simulink model "Automated_IrrigationControlSystem"  (R2023a)
settings: Solver=VariableStepAuto  StartTime=0.0  StopTime=10  MaxStep=1e-3  RelTol=1e-3
libraries: simulink x2
settings Model: Creator=eslam  LastModifiedBy=eslam

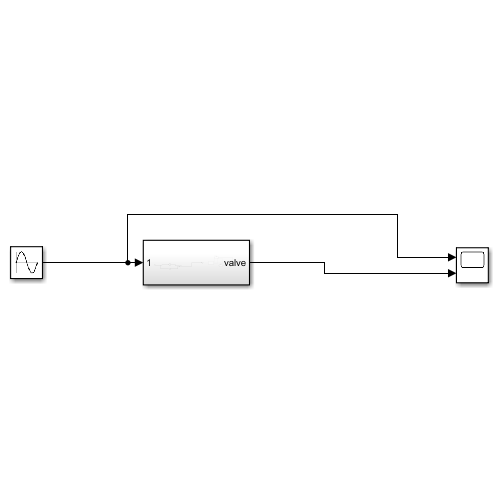
[thumbnail: Simulink's stored preview of the top-level diagram]
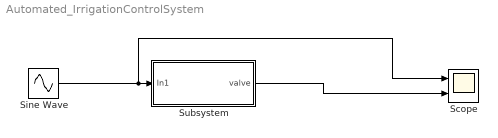
== system Automated_IrrigationControlSystem ==
  Scope : Scope  NumInputPorts=2
  Sine Wave : Sin  Amplitude=88  SampleTime=0
  Subsystem : Subsystem
  wires:
  Sine Wave/1 -> Scope/1, Subsystem/1(In1)
  Subsystem/1(" valve") -> Scope/2

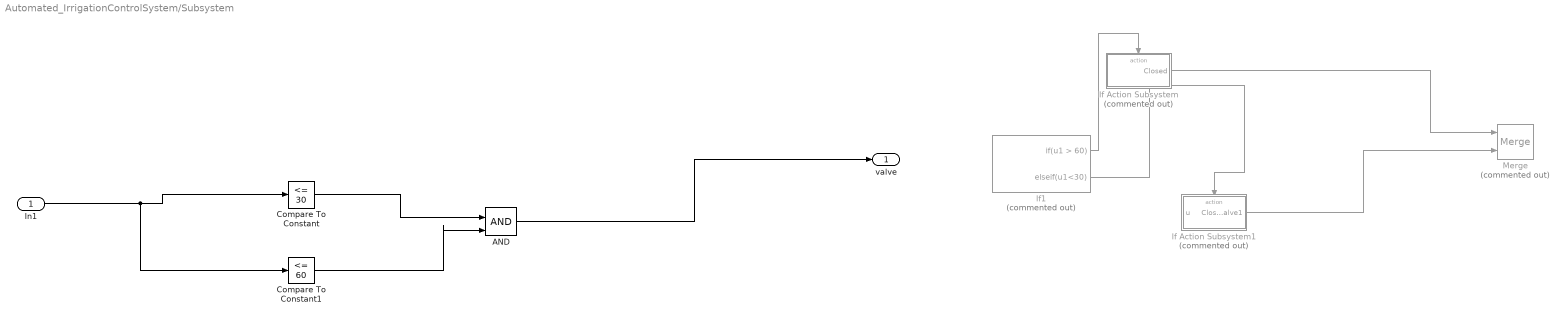
== system Automated_IrrigationControlSystem/Subsystem ==
  In1 : Inport
  AND : Logic  IconShape=distinctive  AllPortsSameDT=off  OutDataTypeStr=boolean
  Compare To Constant : simulink/Logic and Bit Operations/Compare To Constant  relop=<=  const=30  OutDataTypeStr=boolean
  Compare To Constant1 : simulink/Logic and Bit Operations/Compare To Constant  relop=<=  const=60  OutDataTypeStr=boolean
  If Action Subsystem : Subsystem  Commented=on  TreatAsAtomicUnit=on
  If Action Subsystem1 : Subsystem  Commented=on  TreatAsAtomicUnit=on
  If1 : If  Commented=on  IfExpression=u1 > 60  ElseIfExpressions=u1<30  ShowElse=off
  Merge : Merge  Commented=on
  " valve" : Outport
  wires:
  If1/1 -> If Action Subsystem/Action
  If1/2 -> If Action Subsystem1/Action
  If Action Subsystem1/1(Closed valve1) -> Merge/2
  If Action Subsystem/1(Closed) -> Merge/1
  Compare To Constant/1 -> AND/1
  Compare To Constant1/1 -> AND/2
  AND/1 -> " valve"/1
  In1/1 -> Compare To Constant1/1, Compare To Constant/1

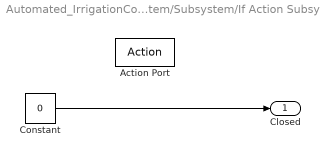
== system Automated_IrrigationControlSystem/Subsystem/If Action Subsystem ==
  Action Port : ActionPort  ActionPortLabel=if(u1 > 60)
  Constant : Constant  Value=0
  Closed : Outport
  wires:
  Constant/1 -> Closed/1

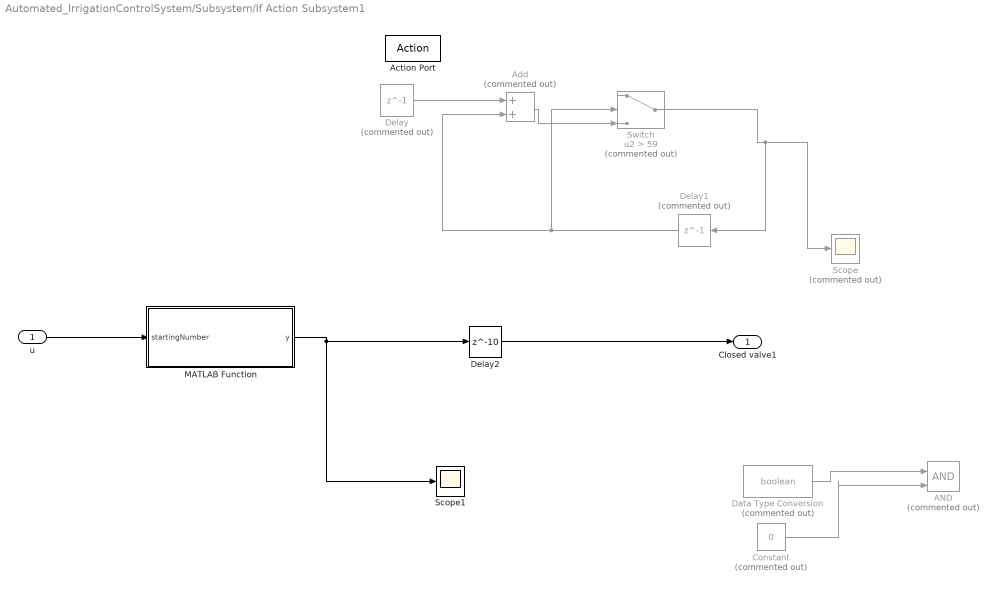
== system Automated_IrrigationControlSystem/Subsystem/If Action Subsystem1 ==
  u : Inport
  Action Port : ActionPort  ActionPortLabel=elseif(u1<30)
  AND : Logic  Commented=on  IconShape=distinctive  AllPortsSameDT=off  OutDataTypeStr=boolean
  Add : Sum  Commented=on
  Constant : Constant  Commented=on  Value=0  OutDataTypeStr=boolean
  Data Type Conversion : DataTypeConversion  Commented=on  OutDataTypeStr=boolean  SaturateOnIntegerOverflow=off  RndMeth=Floor
  Delay : Delay  Commented=on  DelayLength=1
  Delay1 : Delay  Commented=on  DelayLength=1
  Delay2 : Delay  DelayLength=10
  MATLAB Function : MATLAB Function  TreatAsAtomicUnit=on
  Scope : Scope  Commented=on
  Scope1 : Scope
  Switch : Switch  Commented=on  Criteria=u2 > Threshold  Threshold=59  SaturateOnIntegerOverflow=off  InputSameDT=off
  Closed valve1 : Outport
  wires:
  Delay/1 -> Add/1
  Switch/1 -> Delay1/1, Scope/1
  Add/1 -> Switch/3
  Delay1/1 -> Add/2, Switch/2
  u/1 -> MATLAB Function/1(startingNumber)
  Constant/1 -> AND/2
  Data Type Conversion/1 -> AND/1
  MATLAB Function/1(y) -> Delay2/1, Scope1/1
  Delay2/1 -> Closed valve1/1

== matlab function Automated_IrrigationControlSystem/Subsystem/If Action Subsystem1/MATLAB Function ==
  data: startingNumber input; y output
function y = countTo60(startingNumber)
persistent counter;

if isempty(counter)
    counter = startingNumber;
end


if counter <= 60 && counter ~= 0
    counter = counter + 1;
  

end

if counter > 60
    counter = 0;
end

y = counter;
end
